simulink model "question2Sim"  (R2022b)
settings: Solver=VariableStepAuto  StartTime=0.0  StopTime=10.0  RelTol=1e-3
values from neighbouring files (symbols this model uses):
  b2 = 0.4    [question3.m]    (also in question6.m = 10)
  k1 = 6    [question3.m]    (also in question6.m = 2)
  k2 = 4    [question3.m]    (also in question6.m = 2)
  m = 0.1    [question3.m]    (also in question6.m = 20)
settings Model: Creator=adnzw  LastModifiedBy=adnzw

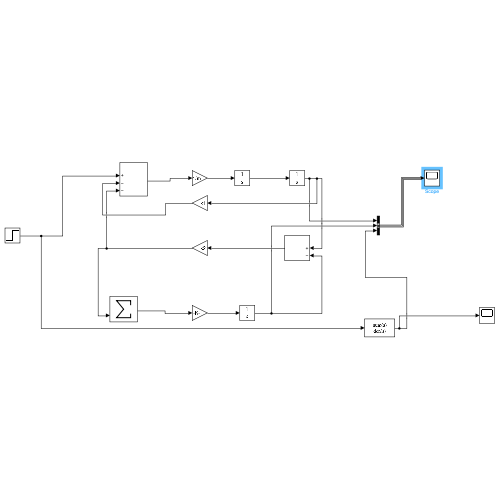
[thumbnail: Simulink's stored preview of the top-level diagram]
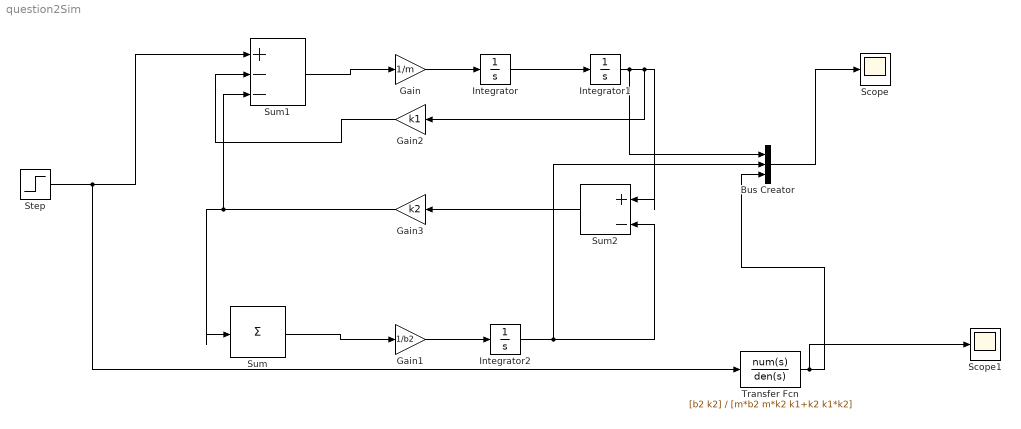
== system question2Sim ==
  Bus Creator : BusCreator  Inputs=3
  Gain : Gain  Gain=1/m
  Gain1 : Gain  Gain=1/b2
  Gain2 : Gain  Gain=k1
  Gain3 : Gain  Gain=k2
  Integrator : Integrator
  Integrator1 : Integrator
  Integrator2 : Integrator
  Scope : Scope
  Scope1 : Scope
  Step : Step  SampleTime=0
  Sum : Sum  Inputs=|+
  Sum1 : Sum  Inputs=|+--
  Sum2 : Sum  Inputs=|+-
  Transfer Fcn : TransferFcn  Numerator=[b2 k2]  Denominator=[m*b2 m*k2 k1+k2 k1*k2]
  wires:
  Sum1/1 -> Gain/1
  Gain/1 -> Integrator/1
  Integrator/1 -> Integrator1/1
  Sum2/1 -> Gain3/1
  Gain1/1 -> Integrator2/1
  Integrator1/1 -> Bus Creator/1, Sum2/1, Gain2/1
  Gain2/1 -> Sum1/2
  Integrator2/1 -> Bus Creator/2, Sum2/2
  Sum/1 -> Gain1/1
  Gain3/1 -> Sum/1, Sum1/3
  Step/1 -> Transfer Fcn/1, Sum1/1
  Bus Creator/1 -> Scope/1
  Transfer Fcn/1 -> Scope1/1, Bus Creator/3
